simulink model "s12_euler_fvm_fanno_ref"  (R2026a)
settings: Solver=FixedStepDiscrete  StopTime=0
model workspace (MAT data in the model file):
  S12_Fanno_DarcyFactor = 0.02
  S12_Fanno_Dt = 0.001
  S12_Fanno_Gamma = 1.4
  S12_Fanno_HydraulicDiameter = 0.1
  S12_Fanno_State = [0  0  0  0  0  0  0  0; 0  0  0  0  0  0  0  0; 0  0  0  0  0  0  0  0]
settings Model: Creator=Jovi  LastModifiedBy=Jovi

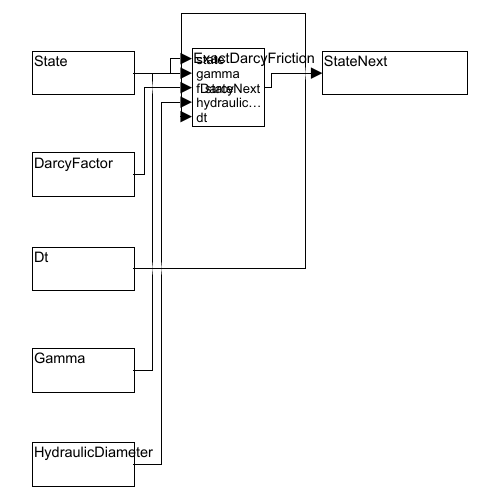
[thumbnail: Simulink's stored preview of the top-level diagram]
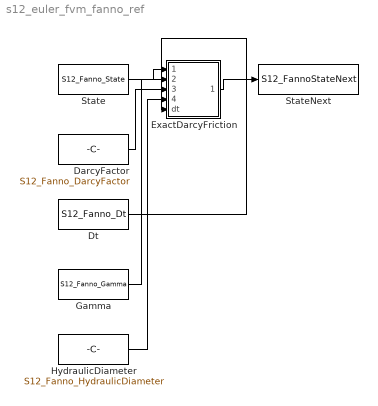
== system s12_euler_fvm_fanno_ref ==
  DarcyFactor : Constant  Value=S12_Fanno_DarcyFactor
  Dt : Constant  Value=S12_Fanno_Dt
  ExactDarcyFriction : MATLAB Function  TreatAsAtomicUnit=on
  Gamma : Constant  Value=S12_Fanno_Gamma
  HydraulicDiameter : Constant  Value=S12_Fanno_HydraulicDiameter
  State : Constant  Value=S12_Fanno_State
  StateNext : ToWorkspace  VariableName=S12_FannoStateNext
  wires:
  ExactDarcyFriction/1(stateNext) -> StateNext/1
  State/1 -> ExactDarcyFriction/1(state)
  Gamma/1 -> ExactDarcyFriction/2(gamma)
  DarcyFactor/1 -> ExactDarcyFriction/3(fDarcy)
  HydraulicDiameter/1 -> ExactDarcyFriction/4(hydraulicDiameter)
  Dt/1 -> ExactDarcyFriction/5(dt)

== matlab function s12_euler_fvm_fanno_ref/ExactDarcyFriction ==
  data: state input; stateNext output; gamma input; fDarcy input; hydraulicDiameter input; dt input
function stateNext = fcn(state, gamma, fDarcy, hydraulicDiameter, dt)
%#codegen
stateNext = state;
if gamma <= 1
    return
end
k = fDarcy / (2 * hydraulicDiameter);
for index = 1:size(state, 2)
    density = state(1, index);
    velocity = state(2, index) / density;
    nextVelocity = velocity / (1 + k * abs(velocity) * dt);
    stateNext(2, index) = density * nextVelocity;
end
end
